simulink model "CMO"  (R2021b)
settings: Solver=VariableStepAuto  StartTime=0.0  StopTime=100  RelTol=1e-3
values from neighbouring files (symbols this model uses):
  m = 5    [L_3.m]    (also in Lab_3_new.m)
  n = 3    [L_3.m]    (also in Lab_3_new.m; st.m = 10)
settings Model: Creator=Анастасия  LastModifiedBy=Анастасия

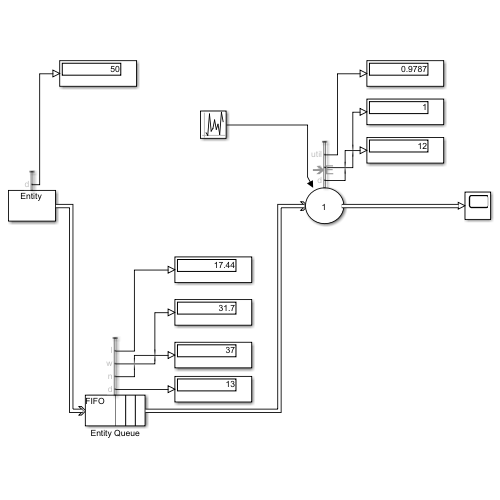
[thumbnail: Simulink's stored preview of the top-level diagram]
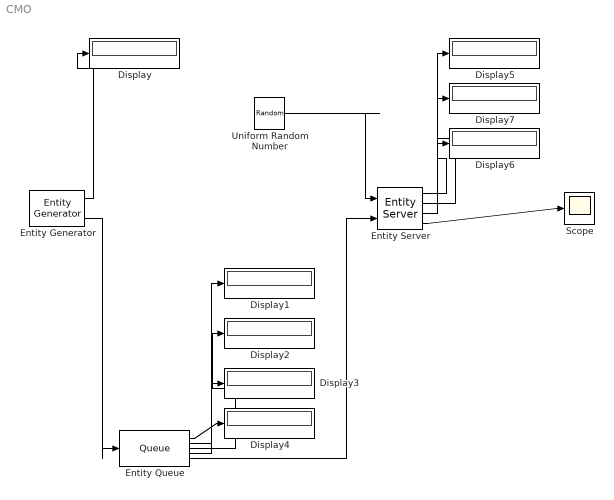
== system CMO ==
  Display{,1..7} (8 alike) : Display
  Entity Generator : EntityGenerator  OutputPortMessageModes=n,m  Period=2  GenerateEntityAtSimulationStart=off  NumberEntitiesDeparted=on  EntityType=Structured  EntityTypeName=Entity
      settings: OutputPortMap=o0,o3
  Entity Queue : Queue  InputPortMessageModes=m  OutputPortMessageModes=n,n,n,n,m  Capacity=inf  NumberEntitiesDeparted=on  NumberEntitiesInBlock=on  AverageWait=on  AverageQueueLength=on
      settings: OutputPortMap=o0,o1,o2,o3,o5
  Entity Server : EntityServer  InputPortMessageModes=n,m  OutputPortMessageModes=n,n,n,m  Capacity=1  ServiceTimeSource=Signal port  NumberEntitiesDeparted=on  NumberEntitiesInBlock=on  Utilization=on
      settings: InputPortMap=u0,u2  OutputPortMap=o0,o1,o5,o9
  Scope : Scope
  Uniform Random Number : UniformRandomNumber  Minimum=5  Maximum=10  SampleTime=0.1
  wires:
  Uniform Random Number/1 -> Entity Server/1
  Entity Server/4 -> Scope/1
  Entity Generator/1 -> Display/1
  Entity Queue/4 -> Display1/1
  Entity Queue/3 -> Display2/1
  Entity Queue/2 -> Display3/1
  Entity Queue/1 -> Display4/1
  Entity Server/3 -> Display5/1
  Entity Server/2 -> Display7/1
  Entity Server/1 -> Display6/1
  Entity Queue/5 -> Entity Server/2
  Entity Generator/2 -> Entity Queue/1
